simulink library "GOcontroll_Moduline_Target"  (R2023b)
settings: Solver=ode45  StartTime=0.0  StopTime=10.0  RelTol=1e-3  EnableMultiTasking=on
PreLoadFcn:
  | compile_gocontroll_mex;
libraries: $bdroot x8, canmsglib x4, simulink x2
(part 3 of 4)

== system GOcontroll_Moduline_Target/Modules/Output Module ==
  Output Module (10 channel) : M-S-Function  FunctionName=sfcn_gocontroll_output_module_10  Parameters=tsamp  mask(10 Channel Output Module){tsamp=0.1, ContrType=GOcontroll Moduline IV, moduleSlot=Moduleslot 1, C12freq=200 Hz, C1func=Disable (output disabled), C2func=Disable (output disabled), C34freq=200 Hz, C3func=Disable (output disabled), C4func=Disable (output disabled), C56freq=200 Hz, C5func=Disable (output disabled), C6func=Disable (output disabled), C78freq=200 Hz, C7func=Disable (output disabled), C8func=Disable (output disabled), C910freq=200 Hz, C9func=Disable (output disabled), C10func=Disable (output disabled)}
      mask prompts: tsamp "Sample time"; ContrType "Controller type"; moduleSlot "Module slot"; C12freq "Frequency"; C1func "Channel 1 function"; C2func "Channel 2 function"; C34freq "Frequency"; C3func "Channel 3 function"; C4func "Channel 4 function"; C56freq "Frequency"; C5func "Channel 5 function"; C6func "Channel 6 function"; C78freq "Frequency"; C7func "Channel 7 function"; C8func "Channel 8 function"; C910freq "Frequency"; C9func "Channel 9 function"; C10func "Channel 10 function"
      mask help:
      | With this function block, you can configure each output of the 10 channel output module (202003xx). During initialization of the controller, the corresponding outputs of the module are set according the settings. During runtime, the value pushed into the block will control the outputs.
      |
      | Sample time:
      | Execution frequency from function block. For proper functioning of the output module, us a sampletime of 100 ms or lower.
      |
      | Module slot:
      | Sets the location of the module slot where the module is physically plugged into.
      |
      | Frequency:
      | In case a duty cycle is used, select the frequency.
      |
      | Function select:
      | Select the desired output configuration for each channel
      mask init:
      | % array with pinID infos
      | moduleSlotInfoStrings = {	'Module Slot 1',  ...\
      | 							'Module Slot 2',  ...\
      | 							'Module Slot 3',  ...\
      | 							'Module Slot 4',  ...\
      | 							'Module Slot 5',  ...\
      | 							'Module Slot 6',  ...\
      | 							'Module Slot 7',  ...\
      | 							'Module Slot 8'};
      | % construct the pinID info string
      | moduleSlotInfoStr = moduleSlotInfoStrings{moduleSlot};
      | 
      | if(moduleSlot == 1 || moduleSlot == 2)
      | 	connectorId = 'A';
      | elseif(moduleSlot == 3 || moduleSlot == 4)
      | 	connectorId = 'B';
      | elseif(moduleSlot == 5 || moduleSlot == 6)
      | 	connectorId = 'D';
      | else
      | 	connectorId = 'E';
      | end
      | 
      | if(ContrType == 1) % Moduline IV
      | 	if(moduleSlot == 1 || moduleSlot == 3 || moduleSlot == 5 || moduleSlot == 7)
      | 		pin1Id = 'Pin 13';
      | 		pin2Id = 'Pin 19';
      | 		pin3Id = 'Pin 12';
      | 		pin4Id = 'Pin 18';
      | 		pin5Id = 'Pin 11';
      | 		pin6Id = 'Pin 17';
      | 		pin7Id = 'Pin 25';
      | 		pin8Id = 'Pin 24';
      | 		pin9Id = 'Pin 5';
      | 		pin10Id = 'Pin 4';
      | 	else
      | 		pin1Id = 'Pin 8';
      | 		pin2Id = 'Pin 14';
      | 		pin3Id = 'Pin 9';
      | 		pin4Id = 'Pin 15';
      | 		pin5Id = 'Pin 10';
      | 		pin6Id = 'Pin 16';
      | 		pin7Id = 'Pin 21';
      | 		pin8Id = 'Pin 22';
      | 		pin9Id = 'Pin 3';
      | 		pin10Id = 'Pin 23';
      | 	end
      | elseif(ContrType == 2 || ContrType == 3) % Moduline mini / Moduline display
      | 	if(moduleSlot == 1 || moduleSlot == 3)
      | 		pin1Id = 'Pin 15';
      | 		pin2Id = 'Pin 23';
      | 		pin3Id = 'Pin 14';
      | 		pin4Id = 'Pin 22';
      | 		pin5Id = 'Pin 13';
      | 		pin6Id = 'Pin 21';
      | 		pin7Id = 'Pin 31';
      | 		pin8Id = 'Pin 30';
      | 		pin9Id = 'Pin 5';
      | 		pin10Id = 'Pin 4';
      | 	else
      | 		pin1Id = 'Pin 10';
      | 		pin2Id = 'Pin 18';
      | 		pin3Id = 'Pin 11';
      | 		pin4Id = 'Pin 19';
      | 		pin5Id = 'Pin 12';
      | 		pin6Id = 'Pin 20';
      | 		pin7Id = 'Pin 27';
      | 		pin8Id = 'Pin 28';
      | 		pin9Id = 'Pin 3';
      | 		pin10Id = 'Pin 29';
      | 	end
      | end
      | 
      | % Create resource keywords to be reserved in resource database
      | modelRTWFields = 	struct('moduleSlot', int2str(moduleSlot),	'C12freq', int2str(C12freq),'C1func', int2str(C1func),'C2func', int2str(C2func),...
      | 																'C34freq', int2str(C34freq),'C3func', int2str(C3func),'C4func', int2str(C4func),...
      | 																'C56freq', int2str(C56freq),'C5func', int2str(C5func),'C6func', int2str(C6func),...
      | 																'C78freq', int2str(C78freq),'C7func', int2str(C7func),'C8func', int2str(C8func),...
      | 																'C910freq', int2str(C910freq),'C9func', int2str(C9func),'C10func', int2str(C10func));
      | 
      | set_param(gcb, 'RTWdata', modelRTWFields);
      mask TypeOptions ContrType: GOcontroll Moduline IV | GOcontroll Moduline Mini | GOcontroll Moduline Display
      mask Callback ContrType:
      | msk = Simulink.Mask.get(gcb);
      | p = msk.getParameter('moduleSlot');
      | 
      | func = get_param(gcb,'ContrType');
      | 
      | if(func == "GOcontroll Moduline IV")
      |     p.TypeOptions = {'Moduleslot 1','Moduleslot 2','Moduleslot 3','Moduleslot 4',...
      |                     'Moduleslot 5','Moduleslot 6','Moduleslot 7','Moduleslot 8'};
      | elseif (func == "GOcontroll Moduline Mini")
      |     p.TypeOptions = {'Moduleslot 1','Moduleslot 2','Moduleslot 3','Moduleslot 4'};
      | elseif (func == "GOcontroll Moduline Display")
      |     p.TypeOptions = {'Moduleslot 1','Moduleslot 2'};
      | end
      mask TypeOptions moduleSlot: Moduleslot 1 | Moduleslot 2 | Moduleslot 3 | Moduleslot 4 | Moduleslot 5 | Moduleslot 6 | Moduleslot 7 | Moduleslot 8
      mask TypeOptions C12freq: 100 Hz | 200 Hz | 500 Hz | 1 kHz
      mask TypeOptions C34freq: 100 Hz | 200 Hz | 500 Hz | 1 kHz
      mask TypeOptions C56freq: 100 Hz | 200 Hz | 500 Hz | 1 kHz
      mask TypeOptions C78freq: 100 Hz | 200 Hz | 500 Hz | 1 kHz
      mask TypeOptions C910freq: 100 Hz | 200 Hz | 500 Hz | 1 kHz
      mask DialogControl Container9 Prompt: Output 1 and 2
      mask DialogControl Container12 Prompt: Output 3 and 4
      mask DialogControl Container13 Prompt: Output 5 and 6
      mask DialogControl Container14 Prompt: Output 7 and 8
      mask DialogControl Container15 Prompt: Output 9 and 10
      mask Display:
      | fprintf('10 Channel Output Module\n%s\n\n Controller Connector: %s', moduleSlotInfoStr,connectorId);%%connectorId
      | port_label('input', 1, pin1Id);
      | port_label('input', 2, pin2Id);
      | port_label('input', 3, pin3Id);
      | port_label('input', 4, pin4Id);
      | port_label('input', 5, pin5Id);
      | port_label('input', 6, pin6Id);
      | port_label('input', 7, pin3Id);
      | port_label('input', 8, pin4Id);
      | port_label('input', 9, pin5Id);
      | port_label('input', 10, pin6Id);
      | text(2, 6, ert_linux_target_version());
  Output Module (6 channel) : M-S-Function  FunctionName=sfcn_gocontroll_output_module  Parameters=tsamp  mask(6 Channel Output Module){tsamp=0.1, ContrType=GOcontroll Moduline IV, moduleSlot=Moduleslot 1, C12freq=200 Hz, C1func=Disable (output disabled), C1cur=4000, C1peakCurrent=1000, C1peakTime=500, C2func=Disable (output disabled), C2cur=4000, C2peakCurrent=1000, C2peakTime=500, C34freq=200 Hz, C3func=Disable (output disabled), C3cur=4000, C3peakCurrent=1000, C3peakTime=500, C4func=Disable (output disabled), C4cur=4000, C4peakCurrent=1000, C4peakTime=500, C56freq=200 Hz, C5func=Disable (output disabled), C5cur=4000, C5peakCurrent=1000, C5peakTime=500, C6func=Disable (output disabled), C6cur=4000, C6peakCurrent=1000, C6peakTime=500}
      mask prompts: tsamp "Sample time"; ContrType "Controller Type"; moduleSlot "Module slot"; C12freq "Frequency"; C1func "Channel 1 function"; C1cur "Channel 1 Imax [mA]"; C1peakCurrent "Peak Current [mA]"; C1peakTime "Peak time [ms]"; C2func "Channel 2 function"; C2cur "Channel 2 Imax [mA]"; C2peakCurrent "Peak Current [mA]"; C2peakTime "Peak time [ms]"; C34freq "Frequency"; C3func "Channel 3 function"; C3cur "Channel 3 Imax [mA]"; C3peakCurrent "Peak Current [mA]"; C3peakTime "Peak time [ms]"; C4func "Channel 4 function"; C4cur "Channel 4 Imax [mA]"; C4peakCurrent "Peak Current [mA]"; C4peakTime "Peak time [ms]"; C56freq "Frequency"; C5func "Channel 5 function"; C5cur "Channel 5 Imax [mA]"; C5peakCurrent "Peak Current [mA]"; C5peakTime "Peak time [ms]"; C6func "Channel 6 function"; C6cur "Channel 6 Imax [mA]"; C6peakCurrent "Peak Current [mA]"; C6peakTime "Peak time [ms]"
      mask help:
      | With this block, you can configure each output of the 6 channel output module (202002xx). During initialization of the controller, the corresponding outputs of the module are set according the settings. During runtime, the value pushed into the block will control the outputs.
      |
      | Sample time:
      | Execution frequency from function block. For proper functioning of the output module, us a sampletime of 100 ms or lower.
      |
      | Module slot:
      | Sets the location of the module slot where the module is physically plugged into.
      |
      | Frequency:
      | In case a duty cycle is used, select the frequency.
      |
      | Function select:
      | Select the desired output configuration for each channel
      mask init:
      | % array with pinID infos
      | moduleSlotInfoStrings = {	'Module slot 1',  ...\
      | 							'Module slot 2',  ...\
      | 							'Module slot 3',  ...\
      | 							'Module slot 4',  ...\
      | 							'Module slot 5',  ...\
      | 							'Module slot 6',  ...\
      | 							'Module slot 7',  ...\
      | 							'Module slot 8'};
      | % construct the pinID info string
      | moduleSlotInfoStr = moduleSlotInfoStrings{moduleSlot};
      | 
      | if(moduleSlot == 1 || moduleSlot == 2)
      | 	connectorId = 'A';
      | elseif(moduleSlot == 3 || moduleSlot == 4)
      | 	connectorId = 'B';
      | elseif(moduleSlot == 5 || moduleSlot == 6)
      | 	connectorId = 'D';
      | else
      | 	connectorId = 'E';
      | end
      | 
      | if(ContrType == 1) % Moduline IV
      | 	if(moduleSlot == 1 || moduleSlot == 3 || moduleSlot == 5 || moduleSlot == 7)
      | 		pin1Id = 'Pin 13';
      | 		pin2Id = 'Pin 19';
      | 		pin3Id = 'Pin 12';
      | 		pin4Id = 'Pin 18';
      | 		pin5Id = 'Pin 11';
      | 		pin6Id = 'Pin 17';
      | 	else
      | 		pin1Id = 'Pin 8';
      | 		pin2Id = 'Pin 14';
      | 		pin3Id = 'Pin 9';
      | 		pin4Id = 'Pin 15';
      | 		pin5Id = 'Pin 10';
      | 		pin6Id = 'Pin 16';
      | 	end
      | elseif(ContrType == 2 || ContrType == 3) % Moduline mini / Moduline Display
      | 	if(moduleSlot == 1 || moduleSlot == 3)
      | 		pin1Id = 'Pin 15';
      | 		pin2Id = 'Pin 23';
      | 		pin3Id = 'Pin 14';
      | 		pin4Id = 'Pin 22';
      | 		pin5Id = 'Pin 13';
      | 		pin6Id = 'Pin 21';
      | 	else
      | 		pin1Id = 'Pin 10';
      | 		pin2Id = 'Pin 18';
      | 		pin3Id = 'Pin 11';
      | 		pin4Id = 'Pin 19';
      | 		pin5Id = 'Pin 12';
      | 		pin6Id = 'Pin 20';
      | 	end
      | end
      | 
      | % Create resource keywords to be reserved in resource database
      | modelRTWFields = 	struct('moduleSlot', int2str(moduleSlot),	'C12freq', int2str(C12freq),...
      | 																'C1func', int2str(C1func),'C2func', int2str(C2func),...
      | 																'C34freq', int2str(C34freq),...
      | 																'C3func', int2str(C3func),'C4func', int2str(C4func),...
      | 																'C56freq', int2str(C56freq),...
      | 																'C5func', int2str(C5func),'C6func', int2str(C6func),...
      | 																'C1cur', int2str(C1cur),'C2cur', int2str(C2cur),...
      | 																'C3cur', int2str(C3cur),'C4cur', int2str(C4cur),...
      | 																'C5cur', int2str(C5cur),'C6cur', int2str(C6cur),...
      | 																'C1peakCurrent', int2str(C1peakCurrent),'C1peakTime', int2str(C1peakTime),...
      | 																'C2peakCurrent', int2str(C2peakCurrent),'C2peakTime', int2str(C2peakTime),...
      | 																'C3peakCurrent', int2str(C3peakCurrent),'C3peakTime', int2str(C3peakTime),...
      | 																'C4peakCurrent', int2str(C4peakCurrent),'C4peakTime', int2str(C4peakTime),...
      | 																'C5peakCurrent', int2str(C5peakCurrent),'C5peakTime', int2str(C5peakTime),...
      | 																'C6peakCurrent', int2str(C6peakCurrent),'C6peakTime', int2str(C6peakTime));
      | 
      | set_param(gcb, 'RTWdata', modelRTWFields);
      mask TypeOptions ContrType: GOcontroll Moduline IV | GOcontroll Moduline Mini | GOcontroll Moduline Display
      mask Callback ContrType:
      | msk = Simulink.Mask.get(gcb);
      | p = msk.getParameter('moduleSlot');
      | 
      | func = get_param(gcb,'ContrType');
      | 
      | if(func == "GOcontroll Moduline IV")
      |     p.TypeOptions = {'Moduleslot 1','Moduleslot 2','Moduleslot 3','Moduleslot 4',...
      |                     'Moduleslot 5','Moduleslot 6','Moduleslot 7','Moduleslot 8'};
      | elseif(func == "GOcontroll Moduline Mini")
      |     p.TypeOptions = {'Moduleslot 1','Moduleslot 2','Moduleslot 3','Moduleslot 4'};
      | elseif (func == "GOcontroll Moduline Display")
      |     p.TypeOptions = {'Moduleslot 1','Moduleslot 2'};
      | end
      mask TypeOptions moduleSlot: Moduleslot 1 | Moduleslot 2 | Moduleslot 3 | Moduleslot 4 | Moduleslot 5 | Moduleslot 6 | Moduleslot 7 | Moduleslot 8
      mask TypeOptions C12freq: 100 Hz | 200 Hz | 500 Hz | 1 kHz | 2 kHz | 5 kHz | 10 kHz
      mask TypeOptions C1func: Disable (output disabled) | Half Bridge duty cycle controlled (0 - 1000) | Low side switch  duty cycle controlled (0 - 1000) | High side switch  duty cycle controlled (0 - 1000) | Low side switch On - Off (0 - 1) | High side switch On - Off (0 - 1) | Peak and hold current mode (Half Bridge) | Frequency output 0 - 500 Hz (0-500)
      mask Callback C1func:
      | func = get_param(gcb,'C1func');
      | p=Simulink.Mask.get(gcb);
      | a=p.getParameter('C1peakCurrent');
      | b=p.getParameter('C1peakTime');
      | c=p.getParameter('C1cur');
      | 
      | if( func == "Peak and hold current mode (Half Bridge)")
      | a.set('Visible','on');
      | b.set('Visible','on');
      | else
      | a.set('Visible','off');
      | b.set('Visible','off');
      | end
      | 
      | if( func == "Disable (output disabled)")
      | c.set('Enabled','off');
      | else
      | c.set('Enabled','on');
      | end
      mask TypeOptions C2func: Disable (output disabled) | Half Bridge duty cycle controlled (0 - 1000) | Low side switch  duty cycle controlled (0 - 1000) | High side switch  duty cycle controlled (0 - 1000) | Low side switch On - Off (0 - 1) | High side switch On - Off (0 - 1) | Peak and hold current mode (Half Bridge) | Frequency output 0 - 500 Hz (0-500)
      mask Callback C2func:
      | func = get_param(gcb,'C2func');
      | p=Simulink.Mask.get(gcb);
      | a=p.getParameter('C2peakCurrent');
      | b=p.getParameter('C2peakTime');
      | c=p.getParameter('C2cur');
      | 
      | if( func == "Peak and hold current mode (Half Bridge)")
      | a.set('Visible','on');
      | b.set('Visible','on');
      | else
      | a.set('Visible','off');
      | b.set('Visible','off');
      | end
      | 
      | if( func == "Disable (output disabled)")
      | c.set('Enabled','off');
      | else
      | c.set('Enabled','on');
      | end
      mask TypeOptions C34freq: 100 Hz | 200 Hz | 500 Hz | 1 kHz | 2 kHz | 5 kHz | 10 kHz
      mask TypeOptions C3func: Disable (output disabled) | Half Bridge duty cycle controlled (0 - 1000) | Low side switch  duty cycle controlled (0 - 1000) | High side switch  duty cycle controlled (0 - 1000) | Low side switch On - Off (0 - 1) | High side switch On - Off (0 - 1) | Peak and hold current mode (Half Bridge) | Frequency output 0 - 500 Hz (0-500)
      mask Callback C3func:
      | func = get_param(gcb,'C3func');
      | p=Simulink.Mask.get(gcb);
      | a=p.getParameter('C3peakCurrent');
      | b=p.getParameter('C3peakTime');
      | c=p.getParameter('C3cur');
      | 
      | if( func == "Peak and hold current mode (Half Bridge)")
      | a.set('Visible','on');
      | b.set('Visible','on');
      | else
      | a.set('Visible','off');
      | b.set('Visible','off');
      | end
      | 
      | if( func == "Disable (output disabled)")
      | c.set('Enabled','off');
      | else
      | c.set('Enabled','on');
      | end
      mask TypeOptions C4func: Disable (output disabled) | Half Bridge duty cycle controlled (0 - 1000) | Low side switch  duty cycle controlled (0 - 1000) | High side switch  duty cycle controlled (0 - 1000) | Low side switch On - Off (0 - 1) | High side switch On - Off (0 - 1) | Peak and hold current mode (Half Bridge) | Frequency output 0 - 500 Hz (0-500)
      mask Callback C4func:
      | func = get_param(gcb,'C4func');
      | p=Simulink.Mask.get(gcb);
      | a=p.getParameter('C4peakCurrent');
      | b=p.getParameter('C4peakTime');
      | c=p.getParameter('C4cur');
      | 
      | if( func == "Peak and hold current mode (Half Bridge)")
      | a.set('Visible','on');
      | b.set('Visible','on');
      | else
      | a.set('Visible','off');
      | b.set('Visible','off');
      | end
      | 
      | if( func == "Disable (output disabled)")
      | c.set('Enabled','off');
      | else
      | c.set('Enabled','on');
      | end
      mask TypeOptions C56freq: 100 Hz | 200 Hz | 500 Hz | 1 kHz | 2 kHz | 5 kHz | 10 kHz
      mask TypeOptions C5func: Disable (output disabled) | Half Bridge duty cycle controlled (0 - 1000) | Low side switch  duty cycle controlled (0 - 1000) | High side switch  duty cycle controlled (0 - 1000) | Low side switch On - Off (0 - 1) | High side switch On - Off (0 - 1) | Peak and hold current mode (Half Bridge) | Frequency output 0 - 500 Hz (0-500)
      mask Callback C5func:
      | func = get_param(gcb,'C5func');
      | p=Simulink.Mask.get(gcb);
      | a=p.getParameter('C5peakCurrent');
      | b=p.getParameter('C5peakTime');
      | c=p.getParameter('C5cur');
      | 
      | if( func == "Peak and hold current mode (Half Bridge)")
      | a.set('Visible','on');
      | b.set('Visible','on');
      | else
      | a.set('Visible','off');
      | b.set('Visible','off');
      | end
      | 
      | if( func == "Disable (output disabled)")
      | c.set('Enabled','off');
      | else
      | c.set('Enabled','on');
      | end
      mask TypeOptions C6func: Disable (output disabled) | Half Bridge duty cycle controlled (0 - 1000) | Low side switch  duty cycle controlled (0 - 1000) | High side switch  duty cycle controlled (0 - 1000) | Low side switch On - Off (0 - 1) | High side switch On - Off (0 - 1) | Peak and hold current mode (Half Bridge) | Frequency output 0 - 500 Hz (0-500)
      mask Callback C6func:
      | func = get_param(gcb,'C6func');
      | p=Simulink.Mask.get(gcb);
      | a=p.getParameter('C6peakCurrent');
      | b=p.getParameter('C6peakTime');
      | c=p.getParameter('C6cur');
      | 
      | if( func == "Peak and hold current mode (Half Bridge)")
      | a.set('Visible','on');
      | b.set('Visible','on');
      | else
      | a.set('Visible','off');
      | b.set('Visible','off');
      | end
      | 
      | if( func == "Disable (output disabled)")
      | c.set('Enabled','off');
      | else
      | c.set('Enabled','on');
      | end
      mask DialogControl Container9 Prompt: Output 1 and 2
      mask DialogControl Container12 Prompt: Output 3 and 4
      mask DialogControl Container13 Prompt: Output 5 and 6
      mask Display:
      | fprintf('6 Channel Output Module\n%s\n\n Controller Connector: %s', moduleSlotInfoStr,connectorId);%%connectorId
      | port_label('input', 1, pin1Id);
      | port_label('input', 2, pin2Id);
      | port_label('input', 3, pin3Id);
      | port_label('input', 4, pin4Id);
      | port_label('input', 5, pin5Id);
      | port_label('input', 6, pin6Id);
      | text(2, 6, ert_linux_target_version());
  Output Module Monitor (6 channel) : M-S-Function  FunctionName=sfcn_gocontroll_output_module_monitor  Parameters=tsamp, moduleSlot, C1duty, C2duty, C3duty, C4duty, C5duty, C6duty  mask(Output Module Monitor){tsamp=0.1, ContrType=GOcontroll Moduline IV, moduleSlot=Moduleslot 1, C1duty=0, C2duty=0, C3duty=0, C4duty=0, C5duty=0, C6duty=0}
      mask prompts: tsamp "Sample time"; ContrType "Controller Type"; moduleSlot "Module Slot"
      mask help:
      | With this function block, you can read parameters from the specified 6 channel output module (202002xx). The block will provide some information about the module such as:
      |
      | Module temperature:
      | The temperature in degrees from the output module.
      |
      | Module ground shift
      | In case the ground connection of the module is poor, the power ground is shifted. The value gives the ground difference in mV and schould be beneath 50 mV
      |
      | Module supply voltage
      | The measured supply voltage of the module in mV. This output only works for hardware version 7 and above, gives off 0 otherwise.
      |
      | Channel current
      | The current from each channel is measured and given in mA. If the ouput is configured as high side, the result will be positive. If the ouput is configured as low side, the value will be negative
      |
      | Channel duty cycle
      | This output only appears if the corresponding output module block has a channel in peak and hold mode, and it only works for module firmware 2.1.0 and higher.
      | This output can be used to monitor the actual output duty cycle. This value can then be used to perform extra checks on the output in this mode.
      mask init:
      | % array with pinID infos
      | moduleSlotInfoStrings = {	'Module slot 1',  ...\
      | 							'Module slot 2',  ...\
      | 							'Module slot 3',  ...\
      | 							'Module slot 4',  ...\
      | 							'Module slot 5',  ...\
      | 							'Module slot 6',  ...\
      | 							'Module slot 7',  ...\
      | 							'Module slot 8'};
      | % construct the pinID info string
      | moduleSlotInfoStr = moduleSlotInfoStrings{moduleSlot};
      | 
      | if(moduleSlot == 1 || moduleSlot == 2)
      | connectorId = 'A';
      | elseif(moduleSlot == 3 || moduleSlot == 4)
      | connectorId = 'B';
      | elseif(moduleSlot == 5 || moduleSlot == 6)
      | connectorId = 'D';
      | else
      | connectorId = 'E';
      | end
      | 
      | if(ContrType == 1) % Moduline IV
      | 	if(moduleSlot == 1 || moduleSlot == 3 || moduleSlot == 5 || moduleSlot == 7)
      | 		pin1Id = 'Pin 13';
      | 		pin2Id = 'Pin 19';
      | 		pin3Id = 'Pin 12';
      | 		pin4Id = 'Pin 18';
      | 		pin5Id = 'Pin 11';
      | 		pin6Id = 'Pin 17';
      | 	else
      | 		pin1Id = 'Pin 8';
      | 		pin2Id = 'Pin 14';
      | 		pin3Id = 'Pin 9';
      | 		pin4Id = 'Pin 15';
      | 		pin5Id = 'Pin 10';
      | 		pin6Id = 'Pin 16';
      | 	end
      | elseif(ContrType == 2 || ContrType == 3) % Moduline mini / Moduline display
      | 	if(moduleSlot == 1 || moduleSlot == 3)
      | 		pin1Id = 'Pin 15';
      | 		pin2Id = 'Pin 23';
      | 		pin3Id = 'Pin 14';
      | 		pin4Id = 'Pin 22';
      | 		pin5Id = 'Pin 13';
      | 		pin6Id = 'Pin 17';
      | 	else
      | 		pin1Id = 'Pin 10';
      | 		pin2Id = 'Pin 18';
      | 		pin3Id = 'Pin 11';
      | 		pin4Id = 'Pin 19';
      | 		pin5Id = 'Pin 12';
      | 		pin6Id = 'Pin 20';
      | 	end
      | end
      | 
      | 
      | 
      | % Create resource keywords to be reserved in resource database
      | modelRTWFields = 	struct('moduleSlot', int2str(moduleSlot), 'C1duty', int2str(C1duty), 'C2duty', int2str(C2duty), ...
      |     'C3duty', int2str(C3duty), 'C4duty', int2str(C4duty), 'C5duty', int2str(C5duty), 'C6duty', int2str(C6duty));
      | 
      | set_param(gcb, 'RTWdata', modelRTWFields);
      mask TypeOptions ContrType: GOcontroll Moduline IV | GOcontroll Moduline Mini | GOcontroll Moduline Display
      mask Callback ContrType:
      | msk = Simulink.Mask.get(gcb);
      | p = msk.getParameter('moduleSlot');
      | 
      | func = get_param(gcb,'ContrType');
      | 
      | if(func == "GOcontroll Moduline IV")
      |     p.TypeOptions = {'Moduleslot 1','Moduleslot 2','Moduleslot 3','Moduleslot 4',...
      |                     'Moduleslot 5','Moduleslot 6','Moduleslot 7','Moduleslot 8'};
      | elseif (func == "GOcontroll Moduline Mini")
      |     p.TypeOptions = {'Moduleslot 1','Moduleslot 2','Moduleslot 3','Moduleslot 4'};
      | elseif (func == "GOcontroll Moduline Display")
      |     p.TypeOptions = {'Moduleslot 1','Moduleslot 2'};
      | end
      mask TypeOptions moduleSlot: Moduleslot 1 | Moduleslot 2 | Moduleslot 3 | Moduleslot 4 | Moduleslot 5 | Moduleslot 6 | Moduleslot 7 | Moduleslot 8
      mask Callback moduleSlot:
      | moduleSlot = get_param(gcb, 'moduleSlot');
      | blockPath = split(gcb, '/');
      | output_modules = find_system(blockPath(1), 'RegExp', 'on', 'FollowLinks', 'on', 'MaskType', '6 Channel Output Module');
      | for idx = 1:length(output_modules)
      |     if char(get_param(output_modules, 'moduleSlot')) == char(moduleSlot)
      |         for jdx = 1:6
      |             if get_param(output_modules, sprintf('C%dfunc',jdx)) == "Peak and hold current mode (Half Bridge)"
      |                 set_param(gcb, sprintf('C%dduty',jdx), "1");
      |             else
      |                 set_param(gcb, sprintf('C%dduty',jdx), "0");
      |             end
      |         end
      |         break
      |     else
      |         for jdx = 1:6
      |             set_param(gcb, sprintf('C%dduty',jdx), "0");
      |         end
      |     end
      | end
      mask Display:
      | fprintf('6 Channel Output Module Monitor\n%s\n\n Controller Connector: %s', moduleSlotInfoStr,connectorId);
      | port_label('output', 1, 'Temperature');
      | port_label('output', 2, 'Ground');
      | port_label('output', 3, 'Supply');
      | port_label('output', 4, 'Status');
      | pinIdx = 5;
      | port_label('output', pinIdx, strcat(pin1Id, " current"));
      | pinIdx = pinIdx + 1;
      | if C1duty == 1
      |     port_label('output', pinIdx, strcat(pin1Id, " duty cycle"));
      |     pinIdx = pinIdx + 1;
      | end
      | 
      | port_label('output', pinIdx, strcat(pin2Id, " current"));
      | pinIdx = pinIdx + 1;
      | if C2duty == 1
      |     port_label('output', pinIdx, strcat(pin2Id, " duty cycle"));
      |     pinIdx = pinIdx + 1;
      | end
      | 
      | port_label('output', pinIdx, strcat(pin3Id, " current"));
      | pinIdx = pinIdx + 1;
      | if C3duty == 1
      |     port_label('output', pinIdx, strcat(pin3Id, " duty cycle"));
      |     pinIdx = pinIdx + 1;
      | end
      | 
      | port_label('output', pinIdx, strcat(pin4Id, " current"));
      | pinIdx = pinIdx + 1;
      | if C4duty == 1
      |     port_label('output', pinIdx, strcat(pin4Id, " duty cycle"));
      |     pinIdx = pinIdx + 1;
      | end
      | 
      | port_label('output', pinIdx, strcat(pin5Id, " current"));
      | pinIdx = pinIdx + 1;
      | if C5duty == 1
      |     port_label('output', pinIdx, strcat(pin5Id, " duty cycle"));
      |     pinIdx = pinIdx + 1;
      | end
      | 
      | port_label('output', pinIdx, strcat(pin6Id, " current"));
      | pinIdx = pinIdx + 1;
      | if C6duty == 1
      |     port_label('output', pinIdx, strcat(pin6Id, " duty cycle"));
      |     pinIdx = pinIdx + 1;
      | end
      | 
      | text(2, 6, ert_linux_target_version());

== system GOcontroll_Moduline_Target/Network/MQTT ==

== system GOcontroll_Moduline_Target/Network/TCP ==
  TCP Configure : M-S-Function  FunctionName=sfcn_TCPConfig  mask(TCP Configure){socket_id=id, port=9001, ip='0.0.0.0', socket_mode=Server, remote_port=9002, remote_ip='0.0.0.0', timeout=1000}
      mask prompts: socket_id "Socket id"; port "The port on which to listen/send"; ip "The ip on which to listen/send"; socket_mode "Socket mode:"; remote_port "The port to connect to"; remote_ip "The ip to connect to"; timeout "The connection timeout (ms)"
      mask help:
      | Block to configure a TCP scoket
      |
      | The socket ID should be a unique identifier to link the send and receive blocks to.
      | The name of the actual socket in the C code will be socket_<socket id>, so characters that would not work in a C variable name will not work.
      |
      | Setting the ip to 0.0.0.0 makes the controller accept messages on all interfaces.
      | Set it to the ip of a specific interface to limit this.
      |
      | The socket mode determines whether this socket will listen for a connection or actively try to make one to a given ip and port.
      | Server will wait for something to connect to it, the client will try to connect to a server at the given ip and port
      |
      | Setting the timeout to zero disables the timeout
      |
      | When the disconnect input is true, it will close the current connection if there is one, if there isn't one it will not allow a connection to be made as long as it is true.
      |
      | Outputs whether or not the socket currently has an active connection (true means connnected)
      mask init:
      | if ~is_ip(ip)
      |         error('Entered IP is not valid');
      |     end
      |     if mod(port,1) > 0 || port < intmin('uint16') || port > intmax('uint16')
      |         error('Entered Port is not valid, it should be an integer from 0-65335');
      |     end
      | 
      |     if ~is_ip(remote_ip)
      |         error('Entered remote IP is not valid');
      |     end
      |     if mod(remote_port,1) > 0 || remote_port < intmin('uint16') || remote_port > intmax('uint16')
      |         error('Entered remote Port is not valid, it should be an integer from 0-65335');
      |     end
      | 
      |     if mod(timeout,1) > 0 || timeout < intmin('uint32') || timeout > intmax('uint32')
      |         error('Entered timeout is not valid, it should be an integer from 0-4.294.967.295');
      |     end
      | 
      |     blockPath = split(gcb, '/');
      |     configures = find_system(blockPath(1),'RegExp', 'on','FollowLinks', 'on','MaskType','TCP Configure');
      |     options = cell(1,length(configures));
      |     for idx = 1:length(configures)
      |         options(idx) = get_param(configures(idx),'socket_id');
      |     end
      | 
      |     if length(unique(options)) ~= length(options)
      |         error('Socket id is already in use, set a unique socket id');
      |     end
      | 
      | 	modelRTWFields = struct('port', num2str(port), 'ip', ip, 'socket_id', socket_id, ...
      |         'remote_port', num2str(remote_port), 'remote_ip', remote_ip, 'socket_mode', num2str(socket_mode), 'timeout', num2str(timeout));
      | 
      | 	% Insert modelRTWFields in the I/O block S-Function containing the Tag starting with 'HANcoder_TARGET_'
      | 	HANcoder_TARGET_DataBlock = find_system(gcb, 'RegExp', 'on', 'FollowLinks', 'on', 'LookUnderMasks', 'all', 'BlockType', 'M-S-Function');
      | 	set_param(HANcoder_TARGET_DataBlock{1}, 'RTWdata', modelRTWFields);
      mask TypeOptions socket_mode: Server | Client
      mask Callback socket_mode:
      | mode = get_param(gcb, 'socket_mode');
      | mask = Simulink.Mask.get(gcb);
      | pars = mask.Parameters;
      | if strcmp(mode, 'Server')
      |     pars(5).set('Visible', 'off');
      |     pars(6).set('Visible', 'off');
      | else
      |     pars(5).set('Visible', 'on');
      |     pars(6).set('Visible', 'on');
      | end
      mask Display:
      | if (socket_mode == 1)
      |     fprintf('Configure TCP server\n IP: %s\nPort: %d',ip,port);
      | else
      |     fprintf('Configure TCP client\n IP: %s\nPort: %d\nRemote IP: %s\n Remote port: %d',ip,port,remote_ip,remote_port);
      | end
      | port_label('output', 1, 'connected');
      | port_label('input', 1, 'disconnect');
      | text(2, 6, ert_linux_target_version());
  TCP Receive : S-Function  FunctionName=sfcn_TCPReceive  Parameters=buff_len,socket_mode,socket_id,tsamp  SFunctionDeploymentMode=off  EnableBusSupport=off  mask(TCP Receive){tsamp=-1, socket_id=id, buff_len=1, socket_mode=Server}
      mask prompts: tsamp "Sample time"; socket_id "Socket"; buff_len "Buffer size"
      mask help:
      | Receive all TCP messages on the given socket
      |
      | For every message received this block will call the functions attached to the function call output.
      | In these function calls you can then use the message and message length outputs to process/buffer the received messages.
      |
      | Outputs:
      | function call:
      | Attach to a function call subsystem or something like it to call that function every time a message is received.
      |
      | message:
      | The uint8 vector received from the socket. The length of this vector is likely longer than the actual number of bytes received.
      |
      | message length:
      | The number of bytes actually received, use this to get the actual fresh bytes from the message.
      |
      | Parameters:
      | buffer size:
      | The maximum number of bytes that can be read from the socket in one message, this also determines the width of the message vector.
      mask TypeOptions socket_id: id
      mask Callback socket_id:
      | blockPath = split(gcb, '/');
      | configures = find_system(blockPath(1),'RegExp', 'on','FollowLinks', 'on','MaskType','TCP Configure');
      | mask = Simulink.Mask.get(gcb);
      | pars = mask.Parameters;
      | options = cell(1,length(configures));
      | for idx = 1:length(configures)
      |     options(idx) = get_param(configures(idx),'socket_id');
      | end
      | mask.getParameter('socket_id').TypeOptions = options;
      | for idx = 1:length(configures)
      |     if strcmp(get_param(configures(idx),'socket_id'), get_param(gcb, 'socket_id'))
      |         mode = Simulink.Mask.get(configures{idx}).getParameter('socket_mode').Value;
      |         set_param(gcb, 'socket_mode', mode);
      |     end
      | end
      mask TypeOptions socket_mode: Server | Client
      mask Display:
      | fprintf('TCP Receive\nSocket: %s', socket_id);
      | text(2, 6, ert_linux_target_version());
      | port_label('output', 1, 'function call');
      | port_label('output', 2, 'message');
      | port_label('output', 3, 'message length');
  TCP Send : M-S-Function  FunctionName=sfcn_TCPSend  Parameters=tsamp  mask(TCP Send){socket_id=id, tsamp=1, socket_mode=Server}
      mask prompts: socket_id "Socket"; tsamp "Sample time"
      mask help:
      | Send a TCP message to the chosen sockets connection, whether it be client or server.
      |
      | The Message input should be a uint8 vector, if you end up with a [1xn] or [nx1] matrix, use the reshape block to turn it into a vector.
      mask init:
      | % update RTWdata to call WriteRTW again
      |     modelRTWFields = struct('socket_id', socket_id, 'socket_mode', num2str(socket_mode));
      | 
      |     % Insert modelRTWFields in the I/O block S-Function containing the Tag starting with 'HANcoder_TARGET_'
      |     HANcoder_TARGET_DataBlock = find_system(gcb, 'RegExp', 'on', 'FollowLinks', 'on', 'LookUnderMasks', 'all', 'BlockType', 'M-S-Function');
      |     set_param(HANcoder_TARGET_DataBlock{1}, 'RTWdata', modelRTWFields);
      mask TypeOptions socket_id: id
      mask Callback socket_id:
      | blockPath = split(gcb, '/');
      | configures = find_system(blockPath(1),'RegExp', 'on','FollowLinks', 'on','MaskType','TCP Configure');
      | mask = Simulink.Mask.get(gcb);
      | pars = mask.Parameters;
      | options = cell(1,length(configures));
      | for idx = 1:length(configures)
      |     options(idx) = get_param(configures(idx),'socket_id');
      | end
      | mask.getParameter('socket_id').TypeOptions = options;
      | for idx = 1:length(configures)
      |     if strcmp(get_param(configures(idx),'socket_id'), get_param(gcb, 'socket_id'))
      |         mode = Simulink.Mask.get(configures{idx}).getParameter('socket_mode').Value;
      |         set_param(gcb, 'socket_mode', mode);
      |     end
      | end
      mask TypeOptions socket_mode: Server | Client
      mask Display:
      | fprintf('TCP Send\nSocket: %s',socket_id);
      | port_label('input', 1, 'message');
      | text(2, 6, ert_linux_target_version());

== system GOcontroll_Moduline_Target/Network/UDP ==
  UDP Configure : M-S-Function  FunctionName=sfcn_UDPConfig  mask(UDP Configure){socket_id=id, port=9001, ip='0.0.0.0', broadcast=on}
      mask prompts: socket_id "Socket id"; port "The port on which to listen/send"; ip "The ip on which to listen/send"; broadcast "Allow broadcasting of sent messages"
      mask help:
      | Block to configure a UDP connection
      |
      | The socket ID should be a unique identifier to link the send and receive blocks to.
      | The name of the actual socket in the C code will be socket_<socket id>, so characters that would not work in a C variable name will not work.
      |
      | Setting the ip to 0.0.0.0 makes the controller accept messages on all interfaces.
      | Set it to the ip of a specific interface to limit this.
      |
      | Allowing broadcasting enables you to send messages to a full range of ip addresses, for example:
      | 192.168.255.255 sends messages to 192.168.1.1, 192.168.2.1 ... 192.168.1.2, 192.168.1.3...
      mask init:
      | if broadcast == 0
      |         broadcastStr = "Not broadcasting";
      |     else
      |         broadcastStr = "Broadcasting";
      |     end
      |     if ~is_ip(ip)
      |         error('Entered IP is not valid');
      |     end
      |     if mod(port,1) > 0 || port < intmin('uint16') || port > intmax('uint16')
      |         error('Entered Port is not valid, it should be an integer from 0-65335');
      |     end
      | 
      |     blockPath = split(gcb, '/');
      |     configures = find_system(blockPath(1),'RegExp', 'on','FollowLinks', 'on','MaskType','UDP Configure');
      |     options = cell(1,length(configures));
      |     for idx = 1:length(configures)
      |         options(idx) = get_param(configures(idx),'socket_id');
      |     end
      | 
      |     if length(unique(options)) ~= length(options)
      |         error('Socket id is already in use, set a unique socket id');
      |     end
      | 
      | 	modelRTWFields = struct('port', num2str(port), 'ip', ip, 'broadcast', num2str(broadcast), 'socket_id', socket_id);
      | 
      | 	% Insert modelRTWFields in the I/O block S-Function containing the Tag starting with 'HANcoder_TARGET_'
      | 	HANcoder_TARGET_DataBlock = find_system(gcb, 'RegExp', 'on', 'FollowLinks', 'on', 'LookUnderMasks', 'all', 'BlockType', 'M-S-Function');
      | 	set_param(HANcoder_TARGET_DataBlock{1}, 'RTWdata', modelRTWFields);
      mask Display:
      | fprintf('Configure UDP socket\n IP: %s\nPort: %d\n%s',ip,port,broadcastStr);
      | text(2, 6, ert_linux_target_version());
  UDP Example : Subsystem
  UDP Receive : S-Function  FunctionName=sfcn_UDPReceive  Parameters=buff_len,socket_id,tsamp  SFunctionDeploymentMode=off  EnableBusSupport=off  mask(UDP Receive){tsamp=-1, socket_id=id, buff_len=1}
      mask prompts: tsamp "Sample time"; socket_id "Socket"; buff_len "Buffer size"
      mask help:
      | Receive all UDP messages
      |
      | For every message received this block will call the functions attached to the function call output.
      | In these function calls you can then use the message and message length outputs to process/buffer the received messages.
      |
      | Outputs:
      | function call:
      | Attach to a function call subsystem or something like it to call that function every time a message is received.
      |
      | message:
      | The uint8 vector received from the socket. The length of this vector is likely longer than the actual number of bytes received.
      |
      | message length:
      | The number of bytes actually received, use this to get the actual fresh bytes from the message.
      |
      | Parameters:
      | buffer size:
      | The maximum number of bytes that can be read from the socket in one message, this also determines the width of the message vector.
      mask TypeOptions socket_id: id | led_sinus
      mask Callback socket_id:
      | blockPath = split(gcb, '/');
      | configures = find_system(blockPath(1),'RegExp', 'on','FollowLinks', 'on','MaskType','UDP Configure');
      | mask = Simulink.Mask.get(gcb);
      | pars = mask.Parameters;
      | options = cell(1,length(configures));
      | for idx = 1:length(configures)
      |     options(idx) = get_param(configures(idx),'socket_id');
      | end
      | mask.getParameter('socket_id').TypeOptions = options;
      mask Display:
      | fprintf('UDP Receive');
      | text(2, 6, ert_linux_target_version());
      | port_label('output', 1, 'function call');
      | port_label('output', 2, 'message');
      | port_label('output', 3, 'message length');
  UDP Send : M-S-Function  FunctionName=sfcn_UDPSend  Parameters=tsamp,ip,port  mask(UDP Send){socket_id=id, ip='0.0.0.0', port=9001, tsamp=1}
      mask prompts: socket_id "Socket"; ip "The IP address to send to"; port "The port to send to"; tsamp "Sample time"
      mask help:
      | Send a UDP message to the designated address.
      |
      | The Message input should be a uint8 vector, if you end up with a [1xn] or [nx1] matrix, use the reshape block to turn it into a vector.
      |
      | IP address should be a valid IP address as a string
      |
      | Port should be a within the range of a uint16
      mask init:
      | if ~is_ip(ip)
      |         error('Entered IP is not valid');
      |     end
      |     if mod(port,1) > 0 || port < intmin('uint16') || port > intmax('uint16')
      |         error('Entered Port is not valid, it should be an integer from 0-65335');
      |     end
      |     % update RTWdata to call WriteRTW again
      |     modelRTWFields = struct('port', num2str(port), 'ip', ip, 'socket_id', socket_id);
      | 
      |     % Insert modelRTWFields in the I/O block S-Function containing the Tag starting with 'HANcoder_TARGET_'
      |     HANcoder_TARGET_DataBlock = find_system(gcb, 'RegExp', 'on', 'FollowLinks', 'on', 'LookUnderMasks', 'all', 'BlockType', 'M-S-Function');
      |     set_param(HANcoder_TARGET_DataBlock{1}, 'RTWdata', modelRTWFields);
      mask TypeOptions socket_id: id | led_sinus
      mask Callback socket_id:
      | blockPath = split(gcb, '/');
      | configures = find_system(blockPath(1),'RegExp', 'on','FollowLinks', 'on','MaskType','UDP Configure');
      | mask = Simulink.Mask.get(gcb);
      | pars = mask.Parameters;
      | options = cell(1,length(configures));
      | for idx = 1:length(configures)
      |     options(idx) = get_param(configures(idx),'socket_id');
      | end
      | pars(1).TypeOptions = options;
      mask Display:
      | fprintf('UDP Send\nIP: %s\nPort: %d',ip,port);
      | port_label('input', 1, 'message');
      | text(2, 6, ert_linux_target_version());

== system GOcontroll_Moduline_Target/System/Version ==
  Initialize Function : Subsystem  TreatAsAtomicUnit=on
  tag scope: SwFeature=global, SwFix=global, SwMajor=global
  wires:
  Initialize Function/3(SwFix) -> [SwFix]
  Initialize Function/2(SwFeature) -> [SwFeature]
  Initialize Function/1(SwMajor) -> [SwMajor]

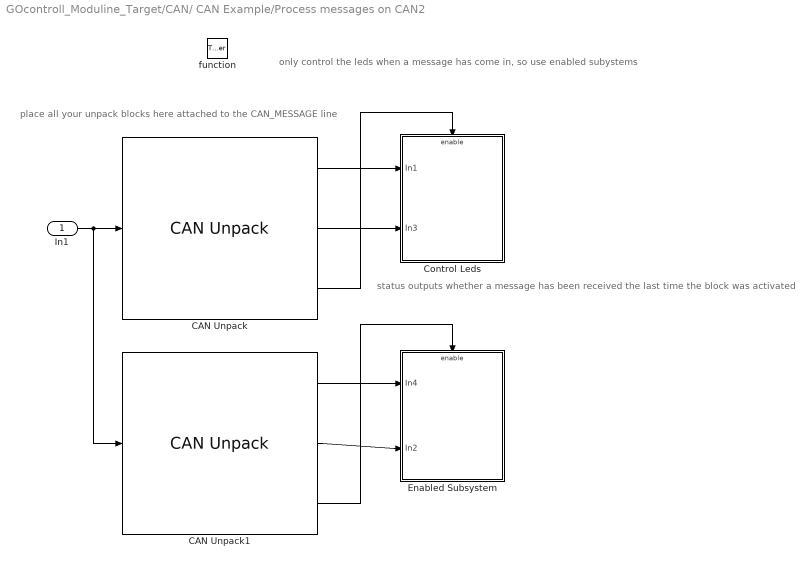
== system GOcontroll_Moduline_Target/CAN/ CAN Example/Process messages on CAN2 ==
  note: only control the leds when a message has come in, so use enabled subystems
  note: place all your unpack blocks here attached to the CAN_MESSAGE line
  note: status outputs whether a message has been received the last time the block was activated
  In1 : Inport
  function : TriggerPort  TriggerType=function-call  VariantControl=(inherit)  OutputDataType=int8
  CAN Unpack : canmsglib/CAN Unpack  MsgList=(none)  MsgName=CAN Msg  MsgIDType=Standard (11-bit identifier)  MsgIdentifier=10  MsgLength=2  SignalInfo={ 'led1', '0', '8', 'LE', 'unsigned', 'Standard', '0', '1', '0', '-Inf', 'Inf'; 'led2', '8', '8', 'LE', 'unsigned', 'Standard', '0', '1', '0', '-Inf', 'Inf' }  IDPort=off  TimestampPort=off  ErrorPort=off  RemotePort=off  LengthPort=off  StatusPort=on  ApplyMinMax=off
      settings: LibrarySourceBlock=embeddedtargetslib/Host Communication/CAN Unpack
  CAN Unpack1 : canmsglib/CAN Unpack  MsgList=(none)  MsgName=CAN Msg  MsgIDType=Standard (11-bit identifier)  MsgIdentifier=11  MsgLength=2  SignalInfo={ 'led3', '0', '8', 'LE', 'unsigned', 'Standard', '0', '1', '0', '-Inf', 'Inf'; 'led4', '8', '8', 'LE', 'unsigned', 'Standard', '0', '1', '0', '-Inf', 'Inf' }  IDPort=off  TimestampPort=off  ErrorPort=off  RemotePort=off  LengthPort=off  StatusPort=on  ApplyMinMax=off
      settings: LibrarySourceBlock=embeddedtargetslib/Host Communication/CAN Unpack
  Control Leds : Subsystem  TreatAsAtomicUnit=on
  Enabled Subsystem : Subsystem  TreatAsAtomicUnit=on
  wires:
  CAN Unpack1/1 -> Enabled Subsystem/1(In4)
  CAN Unpack1/2 -> Enabled Subsystem/2(In2)
  CAN Unpack1/3 -> Enabled Subsystem/Enable
  CAN Unpack/3 -> Control Leds/Enable
  CAN Unpack/1 -> Control Leds/1(In1)
  CAN Unpack/2 -> Control Leds/2(In3)
  In1/1 -> CAN Unpack/1, CAN Unpack1/1

== system GOcontroll_Moduline_Target/Memory store/Diagnostic to memory/Delete all codes for one group ==
  Trigger : TriggerPort  VariantControl=(inherit)  PortDimensions=1
  Delete all DTC fro memory : M-S-Function  FunctionName=sfcn_memory_diagnostic_delete_code  mask(Delete diagnostic codes from memory){}
      mask help:
      | This function block deletes stored codes under the specified diagnostic code type.
      |
      | Sample time:
      | -1 for inherited since this block is a triggered system
      |
      | Diagnostic code type:
      | The type defines the severity of the diagnostic code categorie that is deleted.
      mask init:
      | % Insert modelRTWFields in the I/O block S-Function containing the Tag starting with 'HANcoder_TARGET_'
      | HANcoder_TARGET_DataBlock = find_system(gcb, 'RegExp', 'on', 'FollowLinks', 'on', 'LookUnderMasks', 'all', 'BlockType', 'M-S-Function');
      mask Display:
      | fprintf('Delete all DTCs from memory');
      | text(2, 6, ert_linux_target_version());

== system GOcontroll_Moduline_Target/Memory store/Diagnostic to memory/Delete single DTC code ==
  In1 : Inport
  In2 : Inport  Port=2
  Trigger : TriggerPort  VariantControl=(inherit)
  Delete diagnostic code : M-S-Function  FunctionName=sfcn_memory_diagnostic_delete_single_code  mask(Store diagnostic code to memory){}
      mask help:
      | This function block stores a diagnostic code to memory.
      |
      | Diagnostic code type:
      | The type defines the severity of the diagnostic code.
      |
      | This block should be placed in a triggered subsystem
      mask init:
      | % Insert modelRTWFields in the I/O block S-Function containing the Tag starting with 'HANcoder_TARGET_'
      | HANcoder_TARGET_DataBlock = find_system(gcb, 'RegExp', 'on', 'FollowLinks', 'on', 'LookUnderMasks', 'all', 'BlockType', 'M-S-Function');
      mask Display:
      | fprintf('Delete single DTC from memory');
      | port_label('input', 1, 'SPN');
      | port_label('input', 2, 'FMI');
      | text(2, 6, ert_linux_target_version());
  wires:
  In2/1 -> Delete diagnostic code/2
  In1/1 -> Delete diagnostic code/1

== system GOcontroll_Moduline_Target/Memory store/Diagnostic to memory/Store diagnostic code ==
  Trigger : TriggerPort  VariantControl=(inherit)
  Store DTC code : M-S-Function  FunctionName=sfcn_memory_diagnostic_write_code  mask(Store diagnostic code to memory){spn=spn, fmi=(0) Data valid but above normal operational range, most severe level (3)}
      mask prompts: spn "SPN number"; fmi "Failer Mode Indicator"
      mask help:
      | This function block stores a diagnostic code to memory.
      |
      | Diagnostic code type:
      | The type defines the severity of the diagnostic code.
      |
      | This block should be placed in a triggered subsystem
      mask init:
      | % Create resource keywords to be reserved in resource database
      | modelRTWFields = 	struct(	'spn',int2str(spn),'fmi',int2str(fmi));
      | 
      | % Insert modelRTWFields in the I/O block S-Function containing the Tag starting with 'HANcoder_TARGET_'
      | HANcoder_TARGET_DataBlock = find_system(gcb, 'RegExp', 'on', 'FollowLinks', 'on', 'LookUnderMasks', 'all', 'BlockType', 'M-S-Function');
      | set_param(HANcoder_TARGET_DataBlock{1}, 'RTWdata', modelRTWFields);
      mask Display:
      | fprintf('Store DTC in memory\n SPN: %s\nFMI: %s',spn,fmi);
      | text(2, 6, ert_linux_target_version());
